simulink model "BLDC_model"  (R2012b)
settings: Solver=ode45  StartTime=0.0  StopTime=1  RelTol=1e-3
values from neighbouring files (symbols this model uses):
  f = 12    [Parameters.m]
  J = Jr + Jh    (= 0.0002754438)    [Parameters.m]
  k = 1/(3*R)    (= 0.537634408602)    [Parameters.m]
  k1 = 6.554    [Parameters.m]
  k2 = 2.46    [Parameters.m]
  ki = 25.5e-3*1/2    (= 0.01275)    [Parameters.m]
  kw = 30/(KV*pi)*1/2    (= 0.0127664392854)    [Parameters.m]
  P = 8    [Parameters.m]
  Te = L/R    (= 0.000451612903226)    [Parameters.m]
  tr = cos(EMF_angle/2*pi/180)    [Parameters.m]
  U = 12    [Parameters.m]
settings Model: Creator=botva  LastModifiedBy=botva

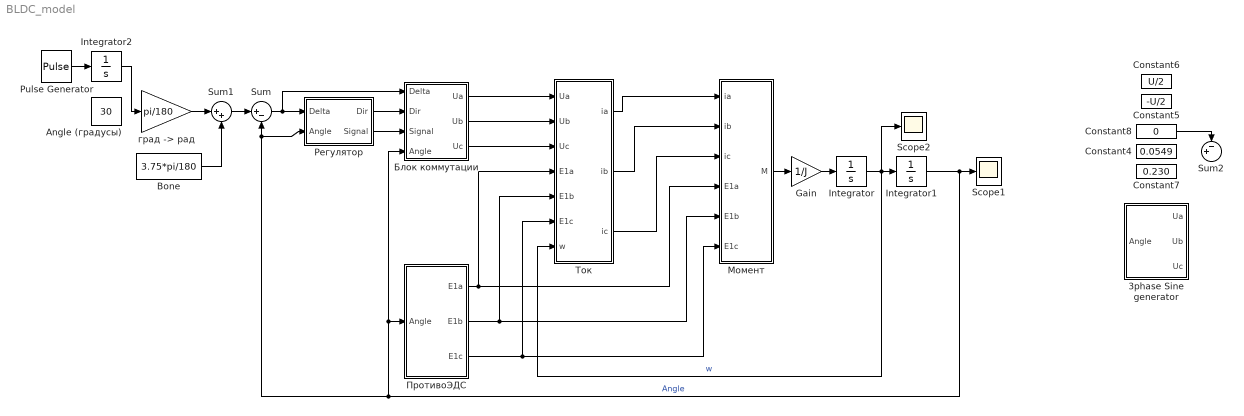
== system BLDC_model ==
  3phase Sine generator : Subsystem
  Angle (градусы) : Constant  Value=30
  Bone : Constant  Value=3.75*pi/180
  Constant4 : Constant  Value=0.0549
  Constant5 : Constant  Value=-U/2
  Constant6 : Constant  Value=U/2
  Constant7 : Constant  Value=0.230
  Constant8 : Constant  Value=0
  Gain : Gain  Gain=1/J
  Integrator : Integrator
  Integrator1 : Integrator  InitialCondition=3.75*pi/180
  Integrator2 : Integrator
  Pulse Generator : DiscretePulseGenerator  PulseType=Time based  Amplitude=360*100  Period=1/f
  Scope1 : Scope
      settings: ShowLegends=on  TimeRange=1  YMin=-0.1  YMax=0.6000000000000001
  Scope2 : Scope
      settings: ShowLegends=on  TimeRange=1  YMin=-0.1  YMax=0.6000000000000001  SaveName=ScopeData2
  Sum : Sum  Inputs=|+-
  Sum1 : Sum  Inputs=|++
  Sum2 : Sum  Inputs=-+|
  Блок коммутации : Subsystem
  Момент : Subsystem
  ПротивоЭДС : Subsystem
  Регулятор : Subsystem
  Ток : Subsystem
  "град -> рад" : Gain  Gain=pi/180
  wires:
  Gain/1 -> Integrator/1
  Integrator/1 -> Scope2/1, Ток/7(w), Integrator1/1  "w"
  Integrator1/1 -> Блок коммутации/4(Angle), ПротивоЭДС/1(Angle), Sum/2, Регулятор/2(Angle), Scope1/1  "Angle"
  ПротивоЭДС/3(E1c) -> Ток/6(E1c), Момент/6(E1c)
  Bone/1 -> Sum1/2
  ПротивоЭДС/2(E1b) -> Ток/5(E1b), Момент/5(E1b)
  Блок коммутации/1(Ua) -> Ток/1(Ua)
  Блок коммутации/2(Ub) -> Ток/2(Ub)
  Блок коммутации/3(Uc) -> Ток/3(Uc)
  Pulse Generator/1 -> Integrator2/1
  Integrator2/1 -> "град -> рад"/1
  Constant8/1 -> Sum2/1
  ПротивоЭДС/1(E1a) -> Ток/4(E1a), Момент/4(E1a)
  Sum/1 -> Регулятор/1(Delta), Блок коммутации/1(Delta)
  "град -> рад"/1 -> Sum1/1
  Регулятор/1(Dir) -> Блок коммутации/2(Dir)
  Sum1/1 -> Sum/1
  Регулятор/2(Signal) -> Блок коммутации/3(Signal)
  Ток/1(ia) -> Момент/1(ia)
  Ток/2(ib) -> Момент/2(ib)
  Ток/3(ic) -> Момент/3(ic)
  Момент/1(M) -> Gain/1

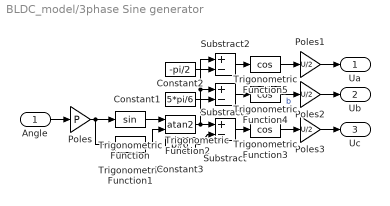
== system BLDC_model/3phase Sine generator ==
  Angle : Inport
  Constant1 : Constant  Value=5*pi/6
  Constant2 : Constant  Value=-pi/2
  Constant3 : Constant  Value=pi/6
  Poles : Gain  Gain=P
  Poles1 : Gain  Gain=U/2
  Poles2 : Gain  Gain=U/2
  Poles3 : Gain  Gain=U/2
  Substract : Sum  Inputs=+-
  Substract1 : Sum  Inputs=+-
  Substract2 : Sum  Inputs=+-
  Trigonometric Function : Trigonometry
  Trigonometric Function{1,3..5} (4 alike) : Trigonometry  Operator=cos
  Trigonometric Function2 : Trigonometry  Operator=atan2
  Ua : Outport
  Ub : Outport  Port=2
  Uc : Outport  Port=3
  wires:
  Trigonometric Function4/1 -> Poles2/1  "b"
  Trigonometric Function5/1 -> Poles1/1
  Trigonometric Function3/1 -> Poles3/1
  Poles/1 -> Trigonometric Function1/1, Trigonometric Function/1
  Trigonometric Function/1 -> Trigonometric Function2/1
  Trigonometric Function1/1 -> Trigonometric Function2/2
  Constant3/1 -> Substract/2
  Substract/1 -> Trigonometric Function3/1
  Constant1/1 -> Substract1/2
  Substract1/1 -> Trigonometric Function4/1
  Constant2/1 -> Substract2/2
  Trigonometric Function2/1 -> Substract2/1, Substract1/1, Substract/1
  Substract2/1 -> Trigonometric Function5/1
  Angle/1 -> Poles/1
  Poles3/1 -> Uc/1
  Poles2/1 -> Ub/1
  Poles1/1 -> Ua/1

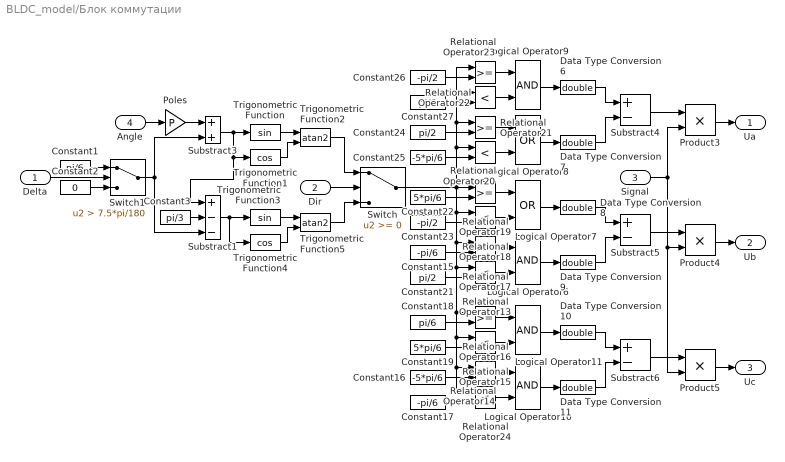
== system BLDC_model/Блок коммутации ==
  Delta : Inport
  Dir : Inport  Port=2
  Signal : Inport  Port=3
  Angle : Inport  Port=4
  Constant1 : Constant  Value=pi/6
  Constant15 : Constant  Value=-pi/6
  Constant16 : Constant  Value=-5*pi/6
  Constant17 : Constant  Value=-pi/6
  Constant18 : Constant  Value=pi/6
  Constant19 : Constant  Value=5*pi/6
  Constant2 : Constant  Value=0
  Constant21 : Constant  Value=pi/2
  Constant22 : Constant  Value=5*pi/6
  Constant23 : Constant  Value=-pi/2
  Constant24 : Constant  Value=pi/2
  Constant25 : Constant  Value=-5*pi/6
  Constant26 : Constant  Value=-pi/2
  Constant27 : Constant  Value=pi/6
  Constant3 : Constant  Value=pi/3
  Data Type Conversion{6..11} (6 alike) : DataTypeConversion  OutDataTypeStr=double
  Logical Operator{6,9..11} (4 alike) : Logic  AllPortsSameDT=off  OutDataTypeStr=boolean
  Logical Operator7 : Logic  Operator=OR  AllPortsSameDT=off  OutDataTypeStr=boolean
  Logical Operator8 : Logic  Operator=OR  AllPortsSameDT=off  OutDataTypeStr=boolean
  Poles : Gain  Gain=P
  Product3 : Product  RndMeth=Zero
  Product4 : Product  RndMeth=Zero
  Product5 : Product  RndMeth=Zero
  Relational Operator{13,15,18,20,22,24} (6 alike) : RelationalOperator  Operator=<  InputSameDT=on
  Relational Operator{14,16..17,19,21,23} (6 alike) : RelationalOperator  InputSameDT=on
  Substract1 : Sum  Inputs=+--
  Substract3 : Sum
  Substract4 : Sum  Inputs=+-
  Substract5 : Sum  Inputs=+-
  Substract6 : Sum  Inputs=+-
  Switch : Switch
  Switch1 : Switch  Criteria=u2 > Threshold  Threshold=7.5*pi/180
  Trigonometric Function : Trigonometry
  Trigonometric Function1 : Trigonometry  Operator=cos
  Trigonometric Function2 : Trigonometry  Operator=atan2
  Trigonometric Function3 : Trigonometry
  Trigonometric Function4 : Trigonometry  Operator=cos
  Trigonometric Function5 : Trigonometry  Operator=atan2
  Ua : Outport
  Ub : Outport  Port=2
  Uc : Outport  Port=3
  wires:
  Trigonometric Function5/1 -> Switch/3
  Substract3/1 -> Substract1/1, Trigonometric Function1/1, Trigonometric Function/1
  Trigonometric Function/1 -> Trigonometric Function2/1
  Trigonometric Function1/1 -> Trigonometric Function2/2
  Relational Operator17/1 -> Logical Operator6/1
  Relational Operator13/1 -> Logical Operator6/2
  Relational Operator19/1 -> Logical Operator7/1
  Relational Operator18/1 -> Logical Operator7/2
  Relational Operator21/1 -> Logical Operator8/1
  Relational Operator20/1 -> Logical Operator8/2
  Relational Operator23/1 -> Logical Operator9/1
  Relational Operator22/1 -> Logical Operator9/2
  Relational Operator24/1 -> Logical Operator10/2
  Relational Operator16/1 -> Logical Operator11/1
  Relational Operator15/1 -> Logical Operator11/2
  Relational Operator14/1 -> Logical Operator10/1
  Substract4/1 -> Product3/1
  Substract6/1 -> Product5/1
  Substract5/1 -> Product4/1
  Data Type Conversion6/1 -> Substract4/1
  Data Type Conversion7/1 -> Substract4/2
  Data Type Conversion8/1 -> Substract5/1
  Data Type Conversion9/1 -> Substract5/2
  Data Type Conversion10/1 -> Substract6/1
  Data Type Conversion11/1 -> Substract6/2
  Product3/1 -> Ua/1
  Product4/1 -> Ub/1
  Product5/1 -> Uc/1
  Constant19/1 -> Relational Operator15/2
  Constant18/1 -> Relational Operator16/2
  Constant21/1 -> Relational Operator13/2
  Constant15/1 -> Relational Operator17/2
  Constant17/1 -> Relational Operator24/2
  Constant16/1 -> Relational Operator14/2
  Constant25/1 -> Relational Operator20/2
  Constant24/1 -> Relational Operator21/2
  Constant23/1 -> Relational Operator18/2
  Constant22/1 -> Relational Operator19/2
  Constant26/1 -> Relational Operator23/2
  Constant27/1 -> Relational Operator22/2
  Logical Operator9/1 -> Data Type Conversion6/1
  Logical Operator8/1 -> Data Type Conversion7/1
  Logical Operator11/1 -> Data Type Conversion10/1
  Logical Operator10/1 -> Data Type Conversion11/1
  Logical Operator7/1 -> Data Type Conversion8/1
  Logical Operator6/1 -> Data Type Conversion9/1
  Switch/1 -> Relational Operator23/1, Relational Operator22/1, Relational Operator21/1, Relational Operator20/1, Relational Operator24/1, Relational Operator14/1, Relational Operator15/1, Relational Operator16/1, Relational Operator13/1, Relational Operator17/1, Relational Operator18/1, Relational Operator19/1
  Trigonometric Function2/1 -> Switch/1
  Dir/1 -> Switch/2
  Signal/1 -> Product3/2, Product4/2, Product5/2
  Trigonometric Function3/1 -> Trigonometric Function5/1
  Trigonometric Function4/1 -> Trigonometric Function5/2
  Substract1/1 -> Trigonometric Function4/1, Trigonometric Function3/1
  Constant3/1 -> Substract1/2
  Delta/1 -> Switch1/2
  Angle/1 -> Poles/1
  Switch1/1 -> Substract3/2, Substract1/3
  Constant1/1 -> Switch1/1
  Constant2/1 -> Switch1/3
  Poles/1 -> Substract3/1

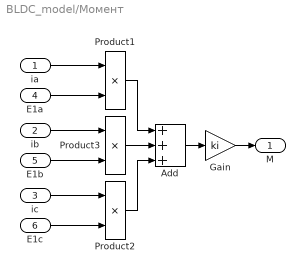
== system BLDC_model/Момент ==
  ia : Inport
  ib : Inport  Port=2
  ic : Inport  Port=3
  E1a : Inport  Port=4
  E1b : Inport  Port=5
  E1c : Inport  Port=6
  Add : Sum  Inputs=+++
  Gain : Gain  Gain=ki
  Product1 : Product  RndMeth=Zero
  Product2 : Product  RndMeth=Zero
  Product3 : Product  RndMeth=Zero
  M : Outport
  wires:
  Gain/1 -> M/1
  Add/1 -> Gain/1
  Product3/1 -> Add/2
  Product1/1 -> Add/1
  Product2/1 -> Add/3
  ia/1 -> Product1/1
  E1a/1 -> Product1/2
  E1c/1 -> Product2/2
  ic/1 -> Product2/1
  E1b/1 -> Product3/2
  ib/1 -> Product3/1

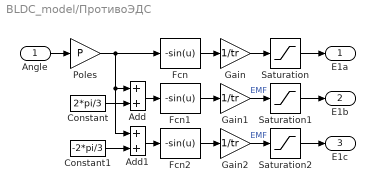
== system BLDC_model/ПротивоЭДС ==
  Angle : Inport
  Add : Sum
  Add1 : Sum
  Constant : Constant  Value=2*pi/3
  Constant1 : Constant  Value=-2*pi/3
  Fcn : Fcn  Expr=-sin(u)
  Fcn1 : Fcn  Expr=-sin(u)
  Fcn2 : Fcn  Expr=-sin(u)
  Gain : Gain  Gain=1/tr
  Gain1 : Gain  Gain=1/tr
  Gain2 : Gain  Gain=1/tr
  Poles : Gain  Gain=P
  Saturation : Saturate  UpperLimit=1  LowerLimit=-1
  Saturation1 : Saturate  UpperLimit=1  LowerLimit=-1
  Saturation2 : Saturate  UpperLimit=1  LowerLimit=-1
  E1a : Outport
  E1b : Outport  Port=2
  E1c : Outport  Port=3
  wires:
  Add/1 -> Fcn1/1
  Constant/1 -> Add/2
  Add1/1 -> Fcn2/1
  Constant1/1 -> Add1/2
  Gain/1 -> Saturation/1
  Fcn/1 -> Gain/1
  Fcn1/1 -> Gain1/1
  Gain1/1 -> Saturation1/1  "EMF"
  Angle/1 -> Poles/1
  Saturation/1 -> E1a/1
  Saturation1/1 -> E1b/1
  Saturation2/1 -> E1c/1
  Poles/1 -> Add1/1, Add/1, Fcn/1
  Fcn2/1 -> Gain2/1
  Gain2/1 -> Saturation2/1  "EMF"

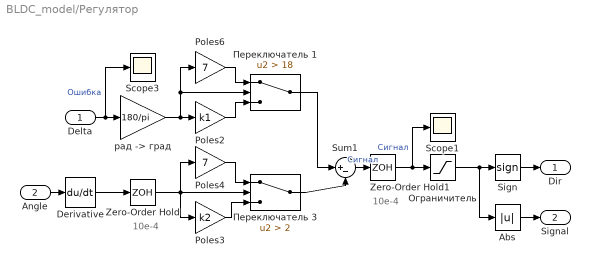
== system BLDC_model/Регулятор ==
  note: 10e-4
  note: 10e-4
  Delta : Inport
  Angle : Inport  Port=2
  Abs : Abs
  Derivative : Derivative
  Poles2 : Gain  Gain=k1
  Poles3 : Gain  Gain=k2
  Poles4 : Gain  Gain=7
  Poles6 : Gain  Gain=7
  Scope1 : Scope
      settings: ShowLegends=on  TimeRange=1  YMin=-0.1  YMax=0.6000000000000001
  Scope3 : Scope
      settings: ShowLegends=on  TimeRange=1  YMin=1.78672  YMax=1.9748  SaveName=ScopeData3
  Sign : Signum
  Sum1 : Sum  Inputs=|+-
  Zero-Order Hold : ZeroOrderHold  SampleTime=10e-4
  Zero-Order Hold1 : ZeroOrderHold  SampleTime=10e-4
  Ограничитель : Saturate  UpperLimit=U/2  LowerLimit=-U/2
  Переключатель 1 : Switch  Criteria=u2 > Threshold  Threshold=18
  Переключатель 3 : Switch  Criteria=u2 > Threshold  Threshold=2  SampleTime=10e-4
  "рад -> град" : Gain  Gain=180/pi
  Dir : Outport
  Signal : Outport  Port=2
  wires:
  Poles2/1 -> Переключатель 1/3
  "рад -> град"/1 -> Poles6/1, Переключатель 1/2, Poles2/1
  Poles6/1 -> Переключатель 1/1
  Ограничитель/1 -> Sign/1, Abs/1
  Abs/1 -> Signal/1
  Sign/1 -> Dir/1
  Delta/1 -> Scope3/1, "рад -> град"/1  "Ошибка"
  Poles3/1 -> Переключатель 3/3
  Poles4/1 -> Переключатель 3/1
  Переключатель 3/1 -> Sum1/2
  Angle/1 -> Derivative/1
  Derivative/1 -> Zero-Order Hold/1
  Zero-Order Hold1/1 -> Scope1/1, Ограничитель/1  "Сигнал"
  Zero-Order Hold/1 -> Poles3/1, Poles4/1, Переключатель 3/2
  Sum1/1 -> Zero-Order Hold1/1  "Сигнал"
  Переключатель 1/1 -> Sum1/1

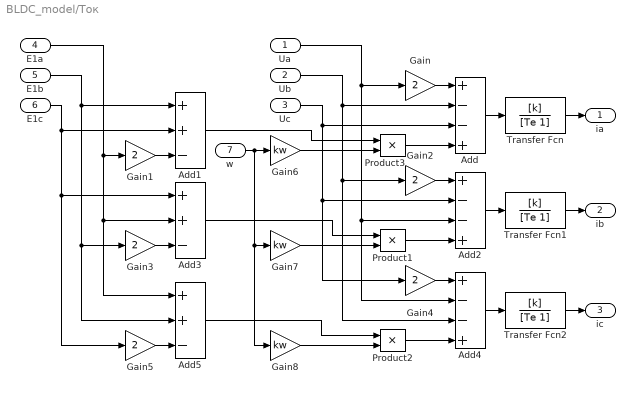
== system BLDC_model/Ток ==
  Ua : Inport
  Ub : Inport  Port=2
  Uc : Inport  Port=3
  E1a : Inport  Port=4
  E1b : Inport  Port=5
  E1c : Inport  Port=6
  w : Inport  Port=7
  Add : Sum  Inputs=+--+
  Add1 : Sum  Inputs=++-
  Add2 : Sum  Inputs=+--+
  Add3 : Sum  Inputs=++-
  Add4 : Sum  Inputs=+--+
  Add5 : Sum  Inputs=++-
  Gain{,1..5} (6 alike) : Gain  Gain=2
  Gain6 : Gain  Gain=kw
  Gain7 : Gain  Gain=kw
  Gain8 : Gain  Gain=kw
  Product1 : Product  RndMeth=Zero
  Product2 : Product  RndMeth=Zero
  Product3 : Product  RndMeth=Zero
  Transfer Fcn : TransferFcn  Numerator=[k]  Denominator=[Te 1]
  Transfer Fcn1 : TransferFcn  Numerator=[k]  Denominator=[Te 1]
  Transfer Fcn2 : TransferFcn  Numerator=[k]  Denominator=[Te 1]
  ia : Outport
  ib : Outport  Port=2
  ic : Outport  Port=3
  wires:
  Add/1 -> Transfer Fcn/1
  Transfer Fcn/1 -> ia/1
  Transfer Fcn1/1 -> ib/1
  Transfer Fcn2/1 -> ic/1
  Product3/1 -> Add/4
  Gain6/1 -> Product3/2
  Gain1/1 -> Add1/3
  Add2/1 -> Transfer Fcn1/1
  Product1/1 -> Add2/4
  Gain7/1 -> Product1/2
  Gain3/1 -> Add3/3
  Add4/1 -> Transfer Fcn2/1
  Uc/1 -> Add/3, Gain4/1, Add2/2
  Ua/1 -> Add4/2, Add2/3, Gain/1
  Ub/1 -> Add/2, Add4/3, Gain2/1
  Product2/1 -> Add4/4
  Gain8/1 -> Product2/2
  Gain5/1 -> Add5/3
  E1b/1 -> Add5/2, Gain3/1, Add1/1
  E1a/1 -> Add5/1, Add3/2, Gain1/1
  E1c/1 -> Gain5/1, Add3/1, Add1/2
  w/1 -> Gain8/1, Gain7/1, Gain6/1
  Add1/1 -> Product3/1
  Add3/1 -> Product1/1
  Add5/1 -> Product2/1
  Gain/1 -> Add/1
  Gain2/1 -> Add2/1
  Gain4/1 -> Add4/1
